simulink model "CompleteModel"  (R2020b)
settings: Solver=ode23t  StartTime=0.0  StopTime=6000  RelTol=1e-3
values from neighbouring files (symbols this model uses):
  alpha_1 = 0.5019    [Data_Parameters_CompleteModel.m]
  alpha_2 = 0.4982    [Data_Parameters_CompleteModel.m]
  Cp = 3200    [Data_Parameters_CompleteModel.m]
  D = [-D2 0 -D4 -2*D5 ... (first row only)    [Data_Parameters_CompleteModel.m]
  d = 1.5e-6    (= 1.5e-06)    [Data_Parameters_CompleteModel.m]
  D2 = 4.438e-14    [Data_Parameters_CompleteModel.m]
  D3 = 1.0024e-14    [Data_Parameters_CompleteModel.m]
  D4 = 3.8e-14    [Data_Parameters_CompleteModel.m]
  D5 = 1.75e-14    [Data_Parameters_CompleteModel.m]
  D_col = 2*A_col/(h_col+w_col)    (= 0.0193548387097)    [Data_Parameters_CompleteModel.m]
  D_L1 = [D_L11 D_L12 D_L13]    [Data_Parameters_CompleteModel.m]
  D_L2 = [D_L21 D_L22 D_L23]    [Data_Parameters_CompleteModel.m]
  D_rec = 2*A_rec/(w_rec+t_rec)    (= 0.00248962655602)    [Data_Parameters_CompleteModel.m]
  F = 96485    [Data_Parameters_CompleteModel.m]
  f_L1 = [f_L11 f_L12 f_L13]    [Data_Parameters_CompleteModel.m]
  f_L2 = [f_L21 f_L22 f_L23]    [Data_Parameters_CompleteModel.m]
  f_value = 58.91    [Data_Parameters_CompleteModel.m]
  H1 = -220000    [Data_Parameters_CompleteModel.m]
  H2 = -64000    [Data_Parameters_CompleteModel.m]
  H4 = -91200    [Data_Parameters_CompleteModel.m]
  H5 = -246800    [Data_Parameters_CompleteModel.m]
  h_col = 0.01    [Data_Parameters_CompleteModel.m]
  k0_1 = 1.6e-6    (= 1.6e-06)    [Data_Parameters_CompleteModel.m]
  k0_2 = 1.5e-4    (= 0.00015)    [Data_Parameters_CompleteModel.m]
  K_con1 = 0.35    [Data_Parameters_CompleteModel.m]
  K_con2 = 0.35    [Data_Parameters_CompleteModel.m]
  K_dec1 = 0.07    [Data_Parameters_CompleteModel.m]
  K_dec2 = 0.07    [Data_Parameters_CompleteModel.m]
  K_E1 = [K_E11 K_E12 K_E13]    [Data_Parameters_CompleteModel.m]
  K_E2 = [K_E21 K_E22 K_E23]    [Data_Parameters_CompleteModel.m]
  K_el = (df^2/(16*CKC))*(porosity^3/(1-porosity)^2)*w_el*t_el    (= 2.96777943925e-13)    [Data_Parameters_CompleteModel.m]
  K_exp1 = 0.7    [Data_Parameters_CompleteModel.m]
  K_exp2 = 0.7    [Data_Parameters_CompleteModel.m]
  K_in1 = 0.5    [Data_Parameters_CompleteModel.m]
  K_in2 = 0.5    [Data_Parameters_CompleteModel.m]
  K_inc1 = 0.68    [Data_Parameters_CompleteModel.m]
  K_inc2 = 0.68    [Data_Parameters_CompleteModel.m]
  K_out1 = 1.0    (= 1)    [Data_Parameters_CompleteModel.m]
  K_out2 = 1.0    (= 1)    [Data_Parameters_CompleteModel.m]
  K_valve1 = 0.06    [Data_Parameters_CompleteModel.m]
  K_valve2 = 0.06    [Data_Parameters_CompleteModel.m]
  Kin = 0.5    [Data_Parameters_CompleteModel.m]
  Kout = 1.0    (= 1)    [Data_Parameters_CompleteModel.m]
  L_col = 0.53    [Data_Parameters_CompleteModel.m]
  L_el = 0.3    [Data_Parameters_CompleteModel.m]
  L_L1 = [L_L11 L_L12 L_L13]    [Data_Parameters_CompleteModel.m]
  L_L2 = [L_L21 L_L22 L_L23]    [Data_Parameters_CompleteModel.m]
  L_rec = 0.02    [Data_Parameters_CompleteModel.m]
  mu = 4.928e-3    (= 0.004928)    [Data_Parameters_CompleteModel.m]
  N = 1    [Data_Parameters_CompleteModel.m]
  N_E1 = [N_E11 N_E12 N_E13]    [Data_Parameters_CompleteModel.m]
  N_E2 = [N_E21 N_E22 N_E23]    [Data_Parameters_CompleteModel.m]
  N_in1 = 2    [Data_Parameters_CompleteModel.m]
  N_in2 = 2    [Data_Parameters_CompleteModel.m]
  N_out1 = 2    [Data_Parameters_CompleteModel.m]
  N_out2 = 2    [Data_Parameters_CompleteModel.m]
  N_valves1 = 3    [Data_Parameters_CompleteModel.m]
  N_valves2 = 3    [Data_Parameters_CompleteModel.m]
  r = 0.04    [Data_Parameters_CompleteModel.m]
  R = 8.31    [Data_Parameters_CompleteModel.m]
  ro = 1354    [Data_Parameters_CompleteModel.m]
  S = 9e-4    (= 0.0009)    [Data_Parameters_CompleteModel.m]
  T = 298    [Data_Parameters_CompleteModel.m]
  t_rec = 0.00125    [Data_Parameters_CompleteModel.m]
  UpAp = 0.47    [Data_Parameters_CompleteModel.m]
  UsAs = 1.31    [Data_Parameters_CompleteModel.m]
  UtAt = 12.69    [Data_Parameters_CompleteModel.m]
  Vcell = 0.0171    [Data_Parameters_CompleteModel.m]
  Vpipe = 1.256e-3    (= 0.001256)    [Data_Parameters_CompleteModel.m]
  Vtank_Anolyte = 45e-6    (= 4.5e-05)    [Data_Parameters_CompleteModel.m]
  Vtank_Catholyte = 55.74e-6    (= 5.574e-05)    [Data_Parameters_CompleteModel.m]
  w_col = 0.3    [Data_Parameters_CompleteModel.m]
  w_rec = 0.3    [Data_Parameters_CompleteModel.m]
undefined symbols (not defined in the file or in its folder): magnitude
(part 1 of 2)
settings Model: Creator=FC_Lab  LastModifiedBy=Alejandro
settings DataIOCC: ReturnWorkspaceOutputs=off
settings DebuggingCC: ArithmeticOperatorsInVariantConditions=warning
settings SFSimCC: SimUseLocalCustomCode=off  CustomCodeUndefinedFunction=UseInterfaceOnly
settings RTWCC: RTWUseLocalCustomCode=off

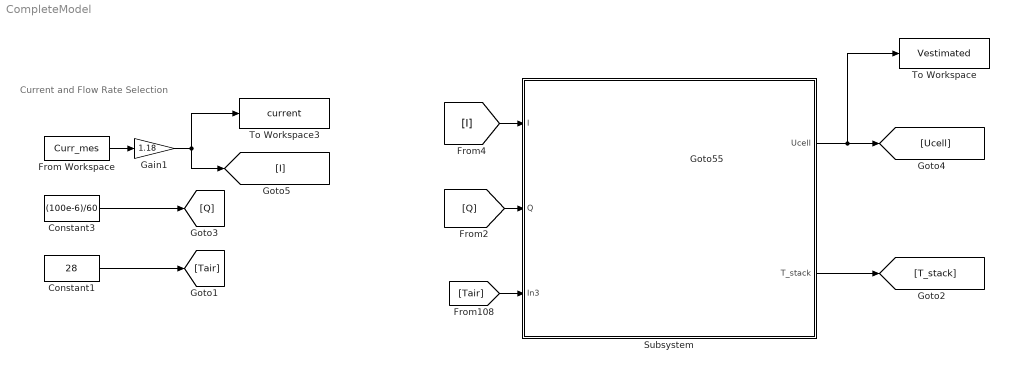
== system CompleteModel ==
  note: Current and Flow Rate Selection
  Constant1 : Constant  Value=28
  Constant3 : Constant  Value=(100e-6)/60
  From Workspace : FromWorkspace  VariableName=Curr_mes
  Gain1 : Gain  Gain=1.18
  Subsystem : Subsystem
      mask Display: image('$imagefile'); % Use "Edit Image" on toolstrip to change.
  To Workspace : ToWorkspace  VariableName=Vestimated  SampleTime=1.0
      settings: Save2DSignal=2-D array (concatenate along first dimension)
  To Workspace3 : ToWorkspace  VariableName=current  SampleTime=1.0
      settings: Save2DSignal=2-D array (concatenate along first dimension)
  wires:
  [I] -> Subsystem/1("I ")
  [Q] -> Subsystem/2(Q)
  [Tair] -> Subsystem/3(In3)
  Subsystem/1(Ucell) -> To Workspace/1, [Ucell]
  Subsystem/2(T_stack) -> [T_stack]
  Constant3/1 -> [Q]
  From Workspace/1 -> Gain1/1
  Gain1/1 -> [I], To Workspace3/1
  Constant1/1 -> [Tair]

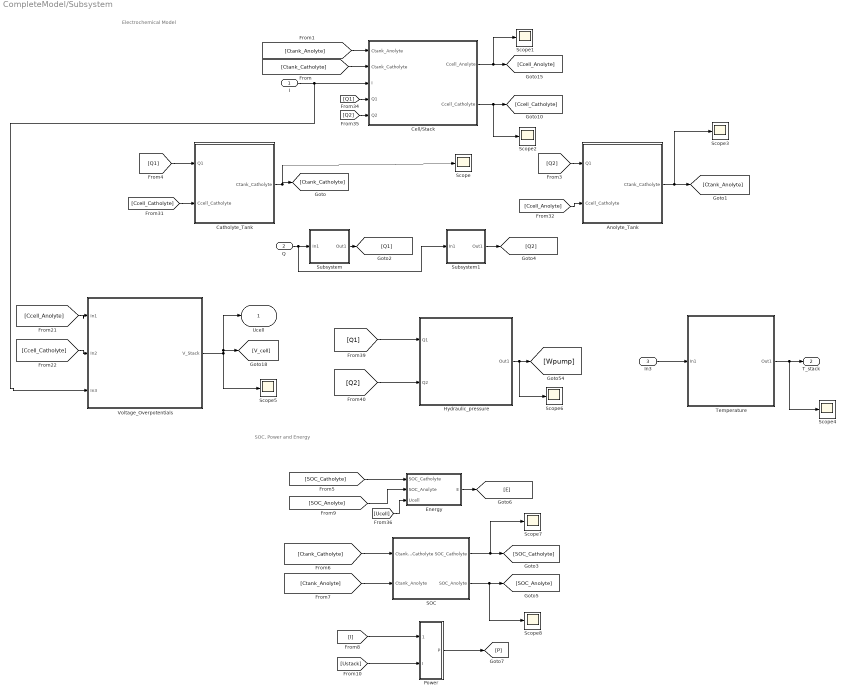
== system CompleteModel/Subsystem ==
  note: SOC, Power and Energy
  note: Electrochemical Model
  "I " : Inport
  Q : Inport  Port=2
  In3 : Inport  Port=3
  Anolyte_Tank : Subsystem  mask(Anolyte tank model){Vtank_Anolyte=55e-6, Ctankini2=5, Ctankini3=395}
      mask help: This subsystem defines the model of the anolyte tank of the redox flow batteries..
      mask Help:
      | The parameters of the block consist on:
      | 
      | Vtank_Anolyte: Volume of the anolye tank (m^3)
      | Ctankini2: Initial concentration of V2 in the anolyte tank (mol/m^3)
      | Ctankini3: Initial concentration of V3 in the anolyte tank (mol/m^3)
      mask DialogControl Container4 Prompt: References
      mask DialogControl Control2 Prompt: 1] Tang, A.; McCann, J.; Bao, J.; Skyllas-Kazacos, M. Investigation of the effect of shunt current on battery efficiency and stack temperature in vanadium redox flow battery.
      mask DialogControl Control3 Prompt: https://doi.org/10.1016/j.jpowsour.2013.05.079.
      mask DialogControl Control4 Prompt: 2] Wei, Z.; Xiong, R.; Lim, T.M.; Meng, S.; Skyllas-Kazacos, M.  Online monitoring of state of charge and1010capacity loss for vanadium redox flow battery based on autoregressive exogenous modeling.
      mask DialogControl Control5 Prompt: https://doi.org/10.1016/j.jpowsour.2018.09.028.
      mask DialogControl Container5 Prompt: Initial concentrations
      mask Display: image('$imagefile'); % Use "Edit Image" on toolstrip to change.
  Catholyte_Tank : Subsystem  mask(Catholyte tank model){Vtank_Catholyte=55e-6, Ctankini4=395, Ctankini5=5}
      mask help: This subsystem defines the model of the catholyte tank of the redox flow batteries..
      mask Help:
      | The parameters of the block consist on:
      | 
      | Vtank_Catholyte: Volume of the catholyte tank (m^3)
      | Ctankini4: Initial concentration of V4 in the cell (mol/m^3)
      | Ctankini5: Initial concentration of V5 in the cell (mol/m^3)
      mask DialogControl Container4 Prompt: References
      mask DialogControl Control2 Prompt: 1] Tang, A.; McCann, J.; Bao, J.; Skyllas-Kazacos, M. Investigation of the effect of shunt current on battery efficiency and stack temperature in vanadium redox flow battery.
      mask DialogControl Control3 Prompt: https://doi.org/10.1016/j.jpowsour.2013.05.079.
      mask DialogControl Control4 Prompt: 2] Wei, Z.; Xiong, R.; Lim, T.M.; Meng, S.; Skyllas-Kazacos, M.  Online monitoring of state of charge and1010capacity loss for vanadium redox flow battery based on autoregressive exogenous modeling.
      mask DialogControl Control5 Prompt: https://doi.org/10.1016/j.jpowsour.2018.09.028.
      mask DialogControl Container5 Prompt: Initial concentrations
      mask Display: image('$imagefile'); % Use "Edit Image" on toolstrip to change.
  Cell/Stack : Subsystem  mask(Cell-Stack model){N=1, Vcell=10e-6, S=1e-4, d=1e-4, Ccellini2=390, Ccellini3=10, Ccellini4=10, Ccellini5=390}
      mask help: This subsystem defines the model of the cell or stack of the redox flow batteries.
      mask Help:
      | The parameters of the block consist on:
      | 
      | N: Number of cells
      | Vcell: Volume of a cell (m^3)
      | S: Electrode surface (m^2)
      | d: Thickness of the membrane (m)
      | Ccellini2: Initial concentration of V2 in the cell (mol/m^3)
      | Ccellini3: Initial concentration of V3 in the cell (mol/m^3)
      | Ccellini4: Initial concentration of V4 in the cell (mol/m^3)
      | Ccellini5: Initial concentration of V5 in the cell (mol/m^3)
      mask DialogControl Container7 Prompt: References
      mask DialogControl Control6 Prompt: 1] Tang, A.; McCann, J.; Bao, J.; Skyllas-Kazacos, M. Investigation of the effect of shunt current on battery efficiency and stack temperature in vanadium redox flow battery.
      mask DialogControl Control4 Prompt: https://doi.org/10.1016/j.jpowsour.2013.05.079.
      mask DialogControl Control7 Prompt: 2] Wei, Z.; Xiong, R.; Lim, T.M.; Meng, S.; Skyllas-Kazacos, M.  Online monitoring of state of charge and1010capacity loss for vanadium redox flow battery based on autoregressive exogenous modeling.
      mask DialogControl Control8 Prompt: https://doi.org/10.1016/j.jpowsour.2018.09.028.
      mask DialogControl Container8 Prompt: Initial concentrations
      mask Display: image('$imagefile'); % Use "Edit Image" on toolstrip to change.
  Energy : Subsystem
  Hydraulic_pressure : Subsystem  mask(Hydraulic losses model){}
      mask help: THis subsystem computes the hydraulic losses due to the pressure of liquids inside the system
      mask DialogControl Container3 Prompt: References
      mask DialogControl Control2 Prompt: Tang,A.;Bao,J.;Skyllas-Kazacos,M.Studies on pressure  losses and flow rate optimization  in  vanadium  redox  flow  battery.
      mask DialogControl Control3 Prompt: https://doi.org/10.1016/j.jpowsour.2013.09.071.
      mask DialogControl Control4 Prompt: Kumar,   S.;    Jayanti,   S.Effect   of   electrode   intrusion   on   pressure   drop   and   electrochemical performance  of  an  all-vanadium  redox  flow  battery.
      mask DialogControl Control5 Prompt: https://doi.org/10.1016/j.jpowsour.2017.06.045.
      mask Display: image('$imagefile'); % Use "Edit Image" on toolstrip to change.
  Power : Subsystem
  SOC : Subsystem
  Scope{,1..8} (9 alike) : Scope
  Subsystem : Subsystem  mask(Pump model){Epump1=1}
      mask help: Model of the pump according to the manufacturer datasheet
      mask Help: Epump: Efficiency of the pump
      mask DialogControl Container4 Prompt: Manufacturer datasheet
      mask DialogControl Control2 Prompt: Model of the pump
      mask Display: image('$imagefile'); % Use "Edit Image" on toolstrip to change.
  Subsystem1 : Subsystem  mask(Pump model){Epump2=1}
      mask help: Model of the pump according to the manufacturer datasheet
      mask Help: Epump2 : Efficiency of the pump
      mask DialogControl Container4 Prompt: Manufacturer datasheet
      mask DialogControl Control2 Prompt: Model of the pump
      mask Display: image('Pump.JPG'); % Use "Edit Image" on toolstrip to change.
  Temperature : Subsystem  mask(Thermal model){}
      mask help: This subsystem presents the thermal model of the redox flow battery.
      mask DialogControl Container4 Prompt: References
      mask DialogControl Control2 Prompt: Tang,   A.;    Ting,   S.;    Bao,   J.;    Skyllas-Kazacos,   M.Thermal   modelling   and   simulation of the  all-vanadium  redox flow  battery.
      mask DialogControl Control3 Prompt: https://doi.org/10.1016/j.jpowsour.2011.11.079.
      mask DialogControl Control4 Prompt: Trovò, A.; Marini, G.; Sutto, A.; Alotto, P.; Giomo, M.; Moro, F.; Guarnieri, M.  Standby thermal model1031of a vanadium redox flow battery stack with crossover and shunt-current effects.
      mask DialogControl Control5 Prompt: https://doi.org/10.1016/j.apenergy.2019.02.067.
      mask DialogControl Control6 Prompt: Tang, A.; Bao, J.; Skyllas-Kazacos, M.  Thermal modelling of battery configuration and self-discharge reactions in vanadium redox flow battery.
      mask DialogControl Control7 Prompt: https://doi.org/10.1016/j.jpowsour.2012.06.052
      mask Display: image('$imagefile'); % Use "Edit Image" on toolstrip to change.
  Voltage_Overpotentials : Subsystem  mask(Voltage and overpotential){E0=1.33, r=0.2, Chini=2000}
      mask help: This block computes the voltage and overpotentials of the cell-stack.
      mask Help:
      | The parameters of the block consist on:
      | 
      | E0: Standard electrode potential (V)
      | r: Ohmic resistance (Ohms)
      | Chini5: Initial concentration of H in the cell (mol/m^3)
      mask DialogControl Container3 Prompt: References
      mask DialogControl Control2 Prompt: (Add text here)
      mask DialogControl Control3 Prompt: (Add text here)
      mask DialogControl Container5 Prompt: Initial concentration
      mask Display: image('$imagefile'); % Use "Edit Image" on toolstrip to change.
  Ucell : Outport
  T_stack : Outport  Port=2
  wires:
  [Ctank_Catholyte] -> Cell/Stack/2(Ctank_Catholyte)
  [Q2] -> Anolyte_Tank/1(Q1)
  [Ccell_Anolyte] -> Anolyte_Tank/2(Ccell_Catholyte)
  [Ustack] -> Power/2(I)
  [SOC_Catholyte] -> Energy/1(SOC_Catholyte)
  Catholyte_Tank/1(Ctank_Catholyte) -> Scope/1, [Ctank_Catholyte]
  Cell/Stack/1(Ccell_Anolyte) -> Scope1/1, [Ccell_Anolyte]
  SOC/2(SOC_Anolyte) -> Scope8/1, [SOC_Anolyte]
  [Q2] -> Cell/Stack/5(Q2)
  [Q1] -> Cell/Stack/4(Q1)
  Energy/1(E) -> [E]
  Cell/Stack/2(Ccell_Catholyte) -> Scope2/1, [Ccell_Catholyte]
  Power/1("P ") -> [P]
  [Ccell_Catholyte] -> Catholyte_Tank/2(Ccell_Catholyte)
  [Ucell] -> Energy/3("Ucell ")
  [Ctank_Anolyte] -> Cell/Stack/1(Ctank_Anolyte)
  [SOC_Anolyte] -> Energy/2(SOC_Anolyte)
  [Ctank_Anolyte] -> SOC/2(Ctank_Anolyte)
  SOC/1(SOC_Catholyte) -> Scope7/1, [SOC_Catholyte]
  [Ctank_Catholyte] -> SOC/1(Ctank_Catholyte)
  [I] -> Power/1(Ustack)
  Anolyte_Tank/1(Ctank_Catholyte) -> Scope3/1, [Ctank_Anolyte]
  "I "/1 -> Voltage_Overpotentials/3(In3), Cell/Stack/3("I ")
  [Q1] -> Catholyte_Tank/1(Q1)
  Subsystem/1(Out1) -> [Q1]
  Subsystem1/1(Out1) -> [Q2]
  Q/1 -> Subsystem1/1(In1), Subsystem/1(In1)
  [Ccell_Anolyte] -> Voltage_Overpotentials/1(In1)
  [Ccell_Catholyte] -> Voltage_Overpotentials/2(In2)
  Voltage_Overpotentials/1(V_Stack) -> Ucell/1, [V_cell], Scope5/1
  [Q1] -> Hydraulic_pressure/1(Q1)
  [Q2] -> Hydraulic_pressure/2(Q2)
  Hydraulic_pressure/1(Out1) -> Scope6/1, [Wpump]
  In3/1 -> Temperature/1(In1)
  Temperature/1(Out1) -> Scope4/1, T_stack/1

== system CompleteModel/Subsystem/Anolyte_Tank ==
  Q1 : Inport
  Ccell_Catholyte : Inport  Port=2
  Gain1 : Gain
  Gain13 : Gain  Gain=1/Vtank_Anolyte
  Integrator Limited4 : Integrator  InitialCondition=[Ctankini2 Ctankini3]  LimitOutput=on  UpperSaturationLimit=400  LowerSaturationLimit=0.001
  Product15 : Product
  Product16 : Product
  Sum12 : Sum  Inputs=|+-
  Ctank_Catholyte : Outport  VectorParamsAs1DForOutWhenUnconnected=off
  wires:
  Gain13/1 -> Integrator Limited4/1
  Sum12/1 -> Gain1/1
  Q1/1 -> Product16/1, Product15/1
  Integrator Limited4/1 -> Ctank_Catholyte/1, Product16/2
  Product15/1 -> Sum12/1
  Product16/1 -> Sum12/2
  Ccell_Catholyte/1 -> Product15/2
  Gain1/1 -> Gain13/1

== system CompleteModel/Subsystem/Catholyte_Tank ==
  Q1 : Inport
  Ccell_Catholyte : Inport  Port=2
  Gain1 : Gain
  Gain13 : Gain  Gain=1/Vtank_Catholyte
  Integrator Limited4 : Integrator  InitialCondition=[Ctankini4 Ctankini5]  LimitOutput=on  UpperSaturationLimit=400  LowerSaturationLimit=0.001
  Product15 : Product
  Product16 : Product
  Sum12 : Sum  Inputs=|+-
  Ctank_Catholyte : Outport  VectorParamsAs1DForOutWhenUnconnected=off
  wires:
  Gain13/1 -> Integrator Limited4/1
  Sum12/1 -> Gain1/1
  Q1/1 -> Product16/1, Product15/1
  Integrator Limited4/1 -> Ctank_Catholyte/1, Product16/2
  Product15/1 -> Sum12/1
  Product16/1 -> Sum12/2
  Ccell_Catholyte/1 -> Product15/2
  Gain1/1 -> Gain13/1

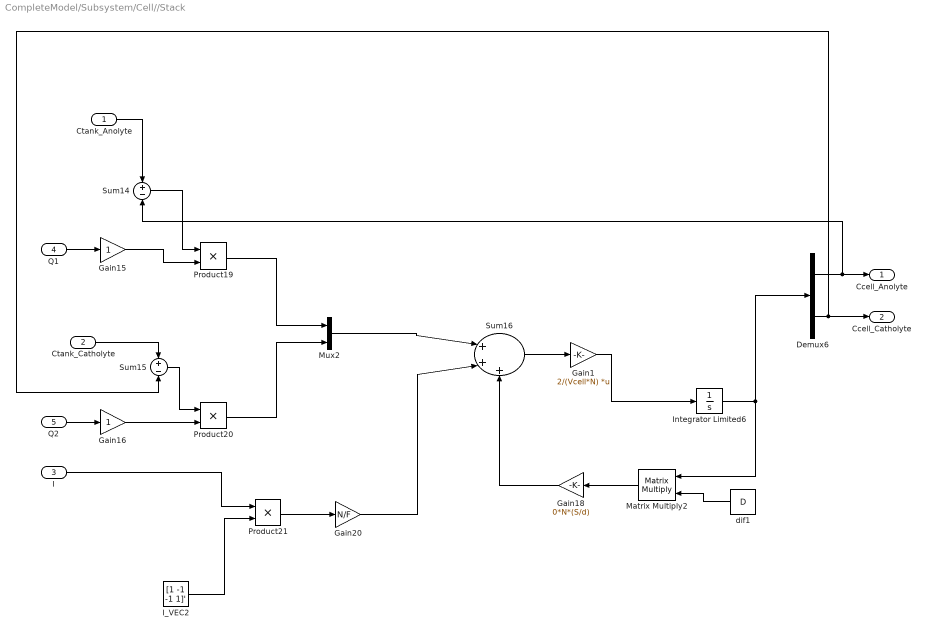
== system CompleteModel/Subsystem/Cell//Stack ==
  Ctank_Anolyte : Inport
  Ctank_Catholyte : Inport  Port=2
  "I " : Inport  Port=3
  Q1 : Inport  Port=4
  Q2 : Inport  Port=5
  Demux6 : Demux  Outputs=2
  Gain1 : Gain  Gain=2/(Vcell*N)  Multiplication=Matrix(K*u)
  Gain15 : Gain
  Gain16 : Gain
  Gain18 : Gain  Gain=0*N*(S/d)
  Gain20 : Gain  Gain=N/F
  I_VEC2 : Constant  Value=[1 -1 -1 1]'
  Integrator Limited6 : Integrator  InitialCondition=[Ccellini2 Ccellini3 Ccellini4 Ccellini5]  LimitOutput=on  UpperSaturationLimit=400  LowerSaturationLimit=0.001
  Matrix Multiply2 : Product  Multiplication=Matrix(*)
  Mux2 : Mux  Inputs=2
  Product19 : Product
  Product20 : Product
  Product21 : Product
  Sum14 : Sum  Inputs=+-
  Sum15 : Sum  Inputs=+-
  Sum16 : Sum  Inputs=|+++
  dif1 : Constant  Value=D
  Ccell_Anolyte : Outport  VectorParamsAs1DForOutWhenUnconnected=off
  Ccell_Catholyte : Outport  Port=2  VectorParamsAs1DForOutWhenUnconnected=off
  wires:
  Gain18/1 -> Sum16/3
  Ctank_Anolyte/1 -> Sum14/1
  Gain20/1 -> Sum16/2
  "I "/1 -> Product21/1
  Integrator Limited6/1 -> Matrix Multiply2/1, Demux6/1
  Sum16/1 -> Gain1/1
  Gain15/1 -> Product19/2
  Sum14/1 -> Product19/1
  Product21/1 -> Gain20/1
  I_VEC2/1 -> Product21/2
  Product19/1 -> Mux2/1
  Sum15/1 -> Product20/1
  Gain16/1 -> Product20/2
  Q1/1 -> Gain15/1
  Matrix Multiply2/1 -> Gain18/1
  dif1/1 -> Matrix Multiply2/2
  Product20/1 -> Mux2/2
  Ctank_Catholyte/1 -> Sum15/1
  Q2/1 -> Gain16/1
  Mux2/1 -> Sum16/1
  Gain1/1 -> Integrator Limited6/1
  Demux6/1 -> Sum14/2, Ccell_Anolyte/1
  Demux6/2 -> Ccell_Catholyte/1, Sum15/2

== system CompleteModel/Subsystem/Energy ==
  SOC_Catholyte : Inport
  SOC_Anolyte : Inport  Port=2
  "Ucell " : Inport  Port=3
  Add : Sum
  Add1 : Sum
  Constant1 : Constant  Value=Vtank_Catholyte
  Constant2 : Constant  Value=F
  Constant3 : Constant  Value=Vtank_Anolyte
  Constant4 : Constant  Value=2000
  Divide11 : Product  Inputs=**
  Divide9 : Product  Inputs=****
  Gain : Gain  Gain=0.5
  Gain1 : Gain  Gain=0.5
  E : Outport  VectorParamsAs1DForOutWhenUnconnected=off
  wires:
  SOC_Anolyte/1 -> Add/2
  Constant2/1 -> Divide9/1
  Divide9/1 -> Divide11/1
  Gain/1 -> Divide9/2
  Add1/1 -> Gain1/1
  Divide11/1 -> E/1
  "Ucell "/1 -> Divide11/2
  Add/1 -> Gain/1
  SOC_Catholyte/1 -> Add/1
  Constant1/1 -> Add1/1
  Constant3/1 -> Add1/2
  Gain1/1 -> Divide9/3
  Constant4/1 -> Divide9/4

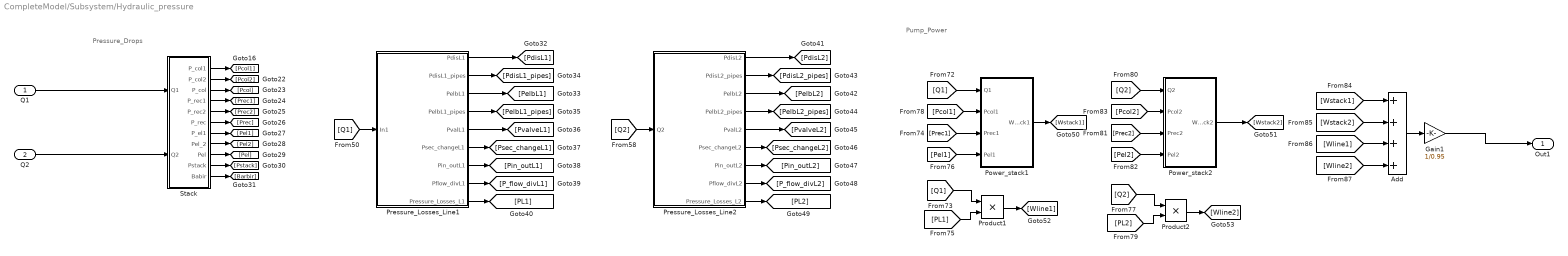
== system CompleteModel/Subsystem/Hydraulic_pressure ==
  note: Pump_Power
  note: Pressure_Drops
  Q1 : Inport
  Q2 : Inport  Port=2
  Add : Sum  Inputs=++++
  Gain1 : Gain  Gain=1/0.95
  Power_stack1 : Subsystem
  Power_stack2 : Subsystem
  Pressure_Losses_Line1 : Subsystem
  Pressure_Losses_Line2 : Subsystem
  Product1 : Product
  Product2 : Product
  Stack : Subsystem
  Out1 : Outport
  wires:
  Pressure_Losses_Line1/7(Pin_outL1) -> [Pin_outL1]
  [Prec1] -> Power_stack1/3(Prec1)
  Pressure_Losses_Line2/2(PdisL2_pipes) -> [PdisL2_pipes]
  [Pcol1] -> Power_stack1/2(Pcol1)
  Stack/2(P_col2) -> [Pcol2]
  Pressure_Losses_Line2/5(PvalL2) -> [PvalveL2]
  Pressure_Losses_Line2/6(Psec_changeL2) -> [Psec_changeL2]
  Power_stack1/1(Wstack1) -> [Wstack1]
  [Q2] -> Pressure_Losses_Line2/1(Q2)
  [Q1] -> Pressure_Losses_Line1/1(In1)
  Add/1 -> Gain1/1
  [Pel1] -> Power_stack1/4(Pel1)
  [Wline2] -> Add/4
  Pressure_Losses_Line2/8(Pflow_divL2) -> [P_flow_divL2]
  Stack/8(Pel_2) -> [Pel2]
  Pressure_Losses_Line2/1(PdisL2) -> [PdisL2]
  Gain1/1 -> Out1/1
  [Wstack1] -> Add/1
  Stack/10(Pstack) -> [Pstack]
  Q1/1 -> Stack/1(Q1)
  Stack/7(P_el1) -> [Pel1]
  Pressure_Losses_Line1/8(Pflow_divL1) -> [P_flow_divL1]
  [Wline1] -> Add/3
  Pressure_Losses_Line2/4(PelbL2_pipes) -> [PelbL2_pipes]
  [PL2] -> Product2/2
  Pressure_Losses_Line1/5(PvalL1) -> [PvalveL1]
  Stack/9(Pel) -> [Pel]
  [Q2] -> Power_stack2/1(Q2)
  Stack/11(Babir) -> [Barbir]
  [PL1] -> Product1/2
  [Q2] -> Product2/1
  [Pel2] -> Power_stack2/4(Pel2)
  Pressure_Losses_Line1/1(PdisL1) -> [PdisL1]
  Pressure_Losses_Line1/4(PelbL1_pipes) -> [PelbL1_pipes]
  Product1/1 -> [Wline1]
  Pressure_Losses_Line1/3(PelbL1) -> [PelbL1]
  Stack/1("P_col1 ") -> [Pcol1]
  [Wstack2] -> Add/2
  Stack/3(P_col) -> [Pcol]
  Stack/6(P_rec) -> [Prec]
  Product2/1 -> [Wline2]
  [Q1] -> Power_stack1/1(Q1)
  Pressure_Losses_Line1/2(PdisL1_pipes) -> [PdisL1_pipes]
  Stack/4(P_rec1) -> [Prec1]
  Power_stack2/1(Wstack2) -> [Wstack2]
  Pressure_Losses_Line1/6(Psec_changeL1) -> [Psec_changeL1]
  [Q1] -> Product1/1
  Q2/1 -> Stack/2(Q2)
  [Prec2] -> Power_stack2/3(Prec2)
  Pressure_Losses_Line2/7(Pin_outL2) -> [Pin_outL2]
  Pressure_Losses_Line2/9(Pressure_Losses_L2) -> [PL2]
  Stack/5(P_rec2) -> [Prec2]
  [Pcol2] -> Power_stack2/2(Pcol2)
  Pressure_Losses_Line2/3(PelbL2) -> [PelbL2]
  Pressure_Losses_Line1/9(Pressure_Losses_L1) -> [PL1]

== system CompleteModel/Subsystem/Power ==
  Ustack : Inport
  I : Inport  Port=2
  Divide11 : Product  Inputs=**
  "P " : Outport  VectorParamsAs1DForOutWhenUnconnected=off
  wires:
  Ustack/1 -> Divide11/1
  Divide11/1 -> "P "/1
  I/1 -> Divide11/2

== system CompleteModel/Subsystem/SOC ==
  Ctank_Catholyte : Inport
  Ctank_Anolyte : Inport  Port=2
  Demux1 : Demux  Outputs=2
  Demux2 : Demux  Outputs=2
  Divide6 : Product  Inputs=*/
  Divide7 : Product  Inputs=*/
  Sum10 : Sum  Inputs=|++
  Sum9 : Sum  Inputs=|++
  SOC_Catholyte : Outport  VectorParamsAs1DForOutWhenUnconnected=off
  SOC_Anolyte : Outport  Port=2  VectorParamsAs1DForOutWhenUnconnected=off
  wires:
  Ctank_Catholyte/1 -> Demux1/1
  Sum10/1 -> Divide7/2
  Demux2/2 -> Divide7/1, Sum10/2
  Sum9/1 -> Divide6/2
  Divide7/1 -> SOC_Anolyte/1
  Demux1/1 -> Sum9/1, Divide6/1
  Demux2/1 -> Sum10/1
  Demux1/2 -> Sum9/2
  Divide6/1 -> SOC_Catholyte/1
  Ctank_Anolyte/1 -> Demux2/1

== system CompleteModel/Subsystem/Subsystem ==
  In1 : Inport
  Gain : Gain  Gain=Epump1
  Out1 : Outport
  wires:
  In1/1 -> Gain/1
  Gain/1 -> Out1/1

== system CompleteModel/Subsystem/Subsystem1 ==
  In1 : Inport
  Gain : Gain  Gain=Epump2
  Out1 : Outport
  wires:
  In1/1 -> Gain/1
  Gain/1 -> Out1/1

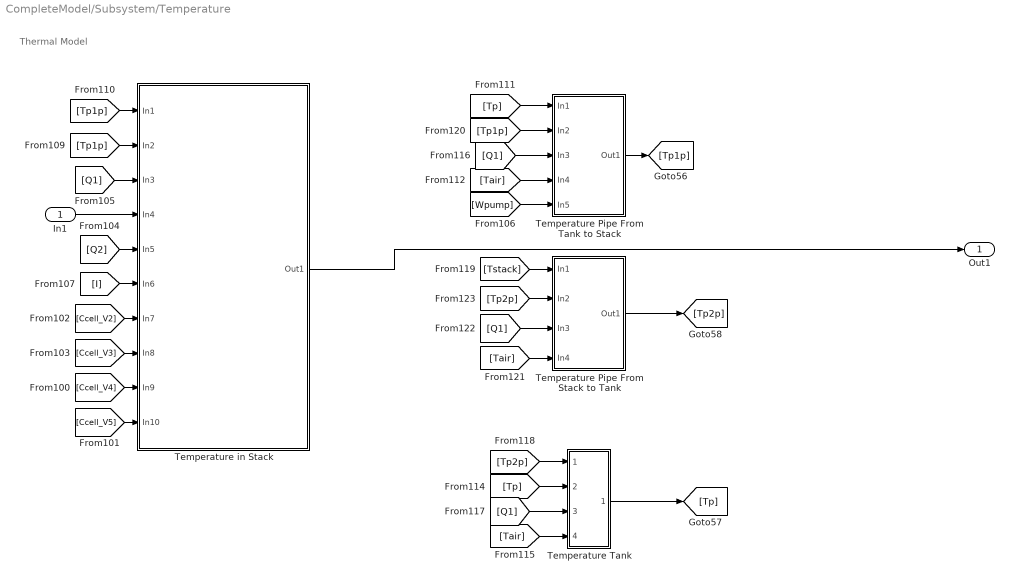
== system CompleteModel/Subsystem/Temperature ==
  note: Thermal Model
  In1 : Inport
  Temperature Tank : Subsystem
  Temperature Pipe From Stack to Tank : Subsystem
  "Temperature Pipe From Tank to Stack " : Subsystem
  Temperature in Stack : Subsystem
  Out1 : Outport
  wires:
  [Ccell_V4] -> Temperature in Stack/9(In9)
  [Q1] -> "Temperature Pipe From Tank to Stack "/3(In3)
  [Ccell_V3] -> Temperature in Stack/8(In8)
  [Tp1p] -> Temperature in Stack/1(In1)
  [Q2] -> Temperature in Stack/5(In5)
  [Tair] -> Temperature Pipe From Stack to Tank/4(In4)
  [Tp2p] -> Temperature Pipe From Stack to Tank/2(In2)
  [Ccell_V2] -> Temperature in Stack/7(In7)
  [Wpump] -> "Temperature Pipe From Tank to Stack "/5(In5)
  [Tp] -> Temperature Tank/2(In2)
  [Q1] -> Temperature Pipe From Stack to Tank/3(In3)
  [Ccell_V5] -> Temperature in Stack/10(In10)
  [Tair] -> "Temperature Pipe From Tank to Stack "/4(In4)
  [Tp2p] -> Temperature Tank/1(In1)
  [Tstack] -> Temperature Pipe From Stack to Tank/1(In1)
  [Q1] -> Temperature Tank/3(In3)
  [Tp1p] -> Temperature in Stack/2(In2)
  [I] -> Temperature in Stack/6(In6)
  [Tair] -> Temperature Tank/4(In4)
  Temperature Pipe From Stack to Tank/1(Out1) -> [Tp2p]
  [Tp1p] -> "Temperature Pipe From Tank to Stack "/2(In2)
  "Temperature Pipe From Tank to Stack "/1(Out1) -> [Tp1p]
  [Tp] -> "Temperature Pipe From Tank to Stack "/1(In1)
  Temperature Tank/1(Out1) -> [Tp]
  [Q1] -> Temperature in Stack/3(In3)
  Temperature in Stack/1(Out1) -> Out1/1
  In1/1 -> Temperature in Stack/4(In4)

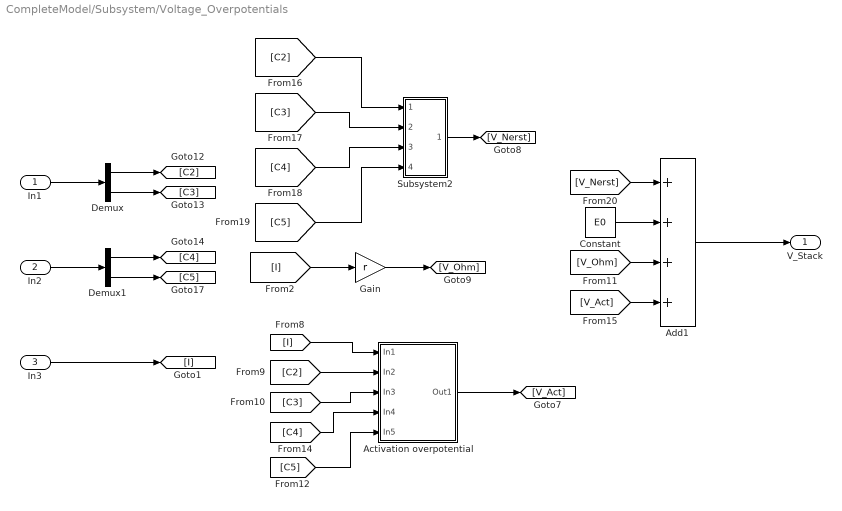
== system CompleteModel/Subsystem/Voltage_Overpotentials ==
  In1 : Inport
  In2 : Inport  Port=2
  In3 : Inport  Port=3
  Activation overpotential : Subsystem
  Add1 : Sum  Inputs=++++
  Constant : Constant  Value=E0
  Demux : Demux  Outputs=2
  Demux1 : Demux  Outputs=2
  Gain : Gain  Gain=r
  Subsystem2 : Subsystem
  V_Stack : Outport
  wires:
  Demux/2 -> [C3]
  Demux1/2 -> [C5]
  Demux1/1 -> [C4]
  Demux/1 -> [C2]
  In1/1 -> Demux/1
  In2/1 -> Demux1/1
  In3/1 -> [I]
  [I] -> Activation overpotential/1(In1)
  Constant/1 -> Add1/2
  Activation overpotential/1(Out1) -> [V_Act]
  [C5] -> Activation overpotential/5(In5)
  [I] -> Gain/1
  Gain/1 -> [V_Ohm]
  [C4] -> Activation overpotential/4(In4)
  [C2] -> Activation overpotential/2(In2)
  [V_Act] -> Add1/4
  [C4] -> Subsystem2/3(In3)
  [V_Ohm] -> Add1/3
  [V_Nerst] -> Add1/1
  [C3] -> Activation overpotential/3(In3)
  Add1/1 -> V_Stack/1
  Subsystem2/1(Out1) -> [V_Nerst]
  [C3] -> Subsystem2/2(In2)
  [C5] -> Subsystem2/4(In4)
  [C2] -> Subsystem2/1(In1)

== system CompleteModel/Subsystem/Hydraulic_pressure/Power_stack1 ==
  Q1 : Inport
  Pcol1 : Inport  Port=2
  Prec1 : Inport  Port=3
  Pel1 : Inport  Port=4
  Add : Sum  Inputs=+++
  Product : Product
  Product1 : Product
  Product2 : Product
  Wstack1 : Outport  VectorParamsAs1DForOutWhenUnconnected=off
  wires:
  Prec1/1 -> Product/2
  Pel1/1 -> Product2/1
  Q1/1 -> Product/1, Product2/2, Product1/1
  Product2/1 -> Add/3
  Add/1 -> Wstack1/1
  Pcol1/1 -> Product1/2
  Product/1 -> Add/2
  Product1/1 -> Add/1

== system CompleteModel/Subsystem/Hydraulic_pressure/Power_stack2 ==
  Q2 : Inport
  Pcol2 : Inport  Port=2
  Prec2 : Inport  Port=3
  Pel2 : Inport  Port=4
  Add : Sum  Inputs=+++
  Product : Product
  Product1 : Product
  Product2 : Product
  Wstack2 : Outport  VectorParamsAs1DForOutWhenUnconnected=off
  wires:
  Prec2/1 -> Product/2
  Pel2/1 -> Product2/1
  Q2/1 -> Product/1, Product2/2, Product1/1
  Product2/1 -> Add/3
  Add/1 -> Wstack2/1
  Pcol2/1 -> Product1/2
  Product/1 -> Add/2
  Product1/1 -> Add/1

== system CompleteModel/Subsystem/Hydraulic_pressure/Pressure_Losses_Line1 ==
  In1 : Inport
  Add : Sum  Inputs=++++++
  Elbows_Losses : Subsystem
  Flow_Division_Losses : Subsystem
  Input_Output_Losses : Subsystem
  Pipes_Distributed_Losses : Subsystem
  Section_Change_Losses : Subsystem
  Valves_Losses : Subsystem
  PdisL1 : Outport  VectorParamsAs1DForOutWhenUnconnected=off
  PdisL1_pipes : Outport  Port=2  VectorParamsAs1DForOutWhenUnconnected=off
  PelbL1 : Outport  Port=3  VectorParamsAs1DForOutWhenUnconnected=off
  PelbL1_pipes : Outport  Port=4  VectorParamsAs1DForOutWhenUnconnected=off
  PvalL1 : Outport  Port=5  VectorParamsAs1DForOutWhenUnconnected=off
  Psec_changeL1 : Outport  Port=6  VectorParamsAs1DForOutWhenUnconnected=off
  Pin_outL1 : Outport  Port=7  VectorParamsAs1DForOutWhenUnconnected=off
  Pflow_divL1 : Outport  Port=8  VectorParamsAs1DForOutWhenUnconnected=off
  Pressure_Losses_L1 : Outport  Port=9  VectorParamsAs1DForOutWhenUnconnected=off
  wires:
  In1/1 -> Elbows_Losses/1(Q1), Valves_Losses/1(Q1), Section_Change_Losses/1(Q1), Input_Output_Losses/1(Q1), Flow_Division_Losses/1(Q1), Pipes_Distributed_Losses/1("Q1 ")
  Section_Change_Losses/1(Psec_change) -> Add/4, Psec_changeL1/1
  Pipes_Distributed_Losses/1(Pdis_L1) -> Add/1, PdisL1/1
  Valves_Losses/1(Pval) -> Add/3, PvalL1/1
  Pipes_Distributed_Losses/2(Pdis_L1_pipes) -> PdisL1_pipes/1
  Elbows_Losses/2(Pelb_pipes) -> PelbL1_pipes/1
  Elbows_Losses/1(Pelb) -> Add/2, PelbL1/1
  Flow_Division_Losses/1(Pflow_div) -> Add/6, Pflow_divL1/1
  Input_Output_Losses/1(Pin_out) -> Add/5, Pin_outL1/1
  Add/1 -> Pressure_Losses_L1/1

== system CompleteModel/Subsystem/Hydraulic_pressure/Pressure_Losses_Line2 ==
  Q2 : Inport
  Add : Sum  Inputs=++++++
  Elbows_Losses : Subsystem
  Flow_Division_Losses : Subsystem
  Input_Output_Losses : Subsystem
  Pipes_Distributed_Losses : Subsystem
  Section_Change_Losses : Subsystem
  Valves_Losses : Subsystem
  PdisL2 : Outport  VectorParamsAs1DForOutWhenUnconnected=off
  PdisL2_pipes : Outport  Port=2  VectorParamsAs1DForOutWhenUnconnected=off
  PelbL2 : Outport  Port=3  VectorParamsAs1DForOutWhenUnconnected=off
  PelbL2_pipes : Outport  Port=4  VectorParamsAs1DForOutWhenUnconnected=off
  PvalL2 : Outport  Port=5  VectorParamsAs1DForOutWhenUnconnected=off
  Psec_changeL2 : Outport  Port=6  VectorParamsAs1DForOutWhenUnconnected=off
  Pin_outL2 : Outport  Port=7  VectorParamsAs1DForOutWhenUnconnected=off
  Pflow_divL2 : Outport  Port=8  VectorParamsAs1DForOutWhenUnconnected=off
  Pressure_Losses_L2 : Outport  Port=9  VectorParamsAs1DForOutWhenUnconnected=off
  wires:
  Q2/1 -> Elbows_Losses/1(Q2), Valves_Losses/1(Q2), Section_Change_Losses/1(Q2), Input_Output_Losses/1(Q2), Flow_Division_Losses/1(Q2), Pipes_Distributed_Losses/1(Q2)
  Section_Change_Losses/1(Psec_change) -> Add/4, Psec_changeL2/1
  Pipes_Distributed_Losses/1(Pdis) -> Add/1, PdisL2/1
  Valves_Losses/1(Pval) -> Add/3, PvalL2/1
  Pipes_Distributed_Losses/2(Pdis_pipes) -> PdisL2_pipes/1
  Elbows_Losses/2(Pelb_pipes) -> PelbL2_pipes/1
  Elbows_Losses/1(Pelb) -> Add/2, PelbL2/1
  Flow_Division_Losses/1(Pflow_div) -> Add/6, Pflow_divL2/1
  Input_Output_Losses/1(Pin_out) -> Add/5, Pin_outL2/1
  Add/1 -> Pressure_Losses_L2/1

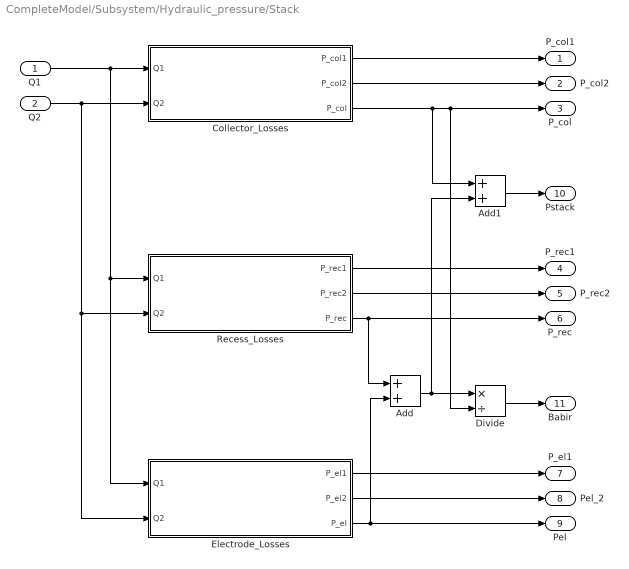
== system CompleteModel/Subsystem/Hydraulic_pressure/Stack ==
  Q1 : Inport
  Q2 : Inport  Port=2
  Add : Sum
  Add1 : Sum
  Collector_Losses : Subsystem
  Divide : Product  Inputs=*/
  Electrode_Losses : Subsystem
  Recess_Losses : Subsystem
  "P_col1 " : Outport  VectorParamsAs1DForOutWhenUnconnected=off
  P_col2 : Outport  Port=2  VectorParamsAs1DForOutWhenUnconnected=off
  P_col : Outport  Port=3  VectorParamsAs1DForOutWhenUnconnected=off
  P_rec1 : Outport  Port=4  VectorParamsAs1DForOutWhenUnconnected=off
  P_rec2 : Outport  Port=5  VectorParamsAs1DForOutWhenUnconnected=off
  P_rec : Outport  Port=6  VectorParamsAs1DForOutWhenUnconnected=off
  P_el1 : Outport  Port=7  VectorParamsAs1DForOutWhenUnconnected=off
  Pel_2 : Outport  Port=8  VectorParamsAs1DForOutWhenUnconnected=off
  Pel : Outport  Port=9  VectorParamsAs1DForOutWhenUnconnected=off
  Pstack : Outport  Port=10  VectorParamsAs1DForOutWhenUnconnected=off
  Babir : Outport  Port=11  VectorParamsAs1DForOutWhenUnconnected=off
  wires:
  Collector_Losses/3(P_col) -> Add1/1, Divide/2, P_col/1
  Recess_Losses/2(P_rec2) -> P_rec2/1
  Q2/1 -> Electrode_Losses/2(Q2), Recess_Losses/2(Q2), Collector_Losses/2(Q2)
  Electrode_Losses/3(P_el) -> Add/2, Pel/1
  Q1/1 -> Electrode_Losses/1(Q1), Recess_Losses/1(Q1), Collector_Losses/1(Q1)
  Electrode_Losses/1(P_el1) -> P_el1/1
  Recess_Losses/3(P_rec) -> Add/1, P_rec/1
  Recess_Losses/1(P_rec1) -> P_rec1/1
  Electrode_Losses/2(P_el2) -> Pel_2/1
  Collector_Losses/2(P_col2) -> P_col2/1
  Collector_Losses/1(P_col1) -> "P_col1 "/1
  Add/1 -> Add1/2, Divide/1
  Divide/1 -> Babir/1
  Add1/1 -> Pstack/1

== system CompleteModel/Subsystem/Temperature/Temperature Tank ==
  In1 : Inport
  In2 : Inport  Port=2
  In3 : Inport  Port=3
  In4 : Inport  Port=4
  Add10 : Sum  Inputs=+-
  Add7 : Sum
  Add9 : Sum  Inputs=+-
  Divide4 : Product  Inputs=**
  Gain14 : Gain  Gain=UtAt
  Gain15 : Gain  Gain=1/(Cp*ro*Vtank_Catholyte)
  Gain16 : Gain  Gain=Cp*ro
  Integrator9 : Integrator  InitialCondition=20
  Out1 : Outport
  wires:
  Divide4/1 -> Add7/1
  Add9/1 -> Gain16/1
  Gain14/1 -> Add7/2
  Add7/1 -> Gain15/1
  Gain15/1 -> Integrator9/1
  In2/1 -> Add10/2, Add9/2
  Gain16/1 -> Divide4/1
  In3/1 -> Divide4/2
  Add10/1 -> Gain14/1
  In1/1 -> Add9/1
  In4/1 -> Add10/1
  Integrator9/1 -> Out1/1

== system CompleteModel/Subsystem/Temperature/Temperature Pipe From Stack to Tank ==
  In1 : Inport
  In2 : Inport  Port=2
  In3 : Inport  Port=3
  In4 : Inport  Port=4
  Add11 : Sum
  Add12 : Sum  Inputs=+-
  Add13 : Sum  Inputs=+-
  Divide5 : Product  Inputs=**
  Gain17 : Gain  Gain=UpAp
  Gain18 : Gain  Gain=1/(Cp*ro*Vpipe)
  Gain19 : Gain  Gain=Cp*ro
  Integrator2 : Integrator
  Out1 : Outport
  wires:
  In2/1 -> Add13/2, Add12/2
  Gain18/1 -> Integrator2/1
  Gain17/1 -> Add11/2
  Add13/1 -> Gain17/1
  Divide5/1 -> Add11/1
  Add11/1 -> Gain18/1
  Add12/1 -> Gain19/1
  Gain19/1 -> Divide5/1
  In1/1 -> Add12/1
  In3/1 -> Divide5/2
  Integrator2/1 -> Out1/1
  In4/1 -> Add13/1

== system CompleteModel/Subsystem/Temperature/Temperature Pipe From Tank to Stack  ==
  In1 : Inport
  In2 : Inport  Port=2
  In3 : Inport  Port=3
  In4 : Inport  Port=4
  In5 : Inport  Port=5
  Add5 : Sum  Inputs=+++
  Add6 : Sum  Inputs=+-
  Add8 : Sum  Inputs=+-
  Divide3 : Product  Inputs=**
  Gain11 : Gain  Gain=UpAp
  Gain12 : Gain  Gain=1/(Cp*ro*Vpipe)
  Gain13 : Gain  Gain=Cp*ro
  Integrator8 : Integrator
  Out1 : Outport
  wires:
  Gain13/1 -> Divide3/1
  In3/1 -> Divide3/2
  Add6/1 -> Gain13/1
  Add8/1 -> Gain11/1
  Gain12/1 -> Integrator8/1
  Divide3/1 -> Add5/1
  In2/1 -> Add8/2, Add6/2
  Gain11/1 -> Add5/2
  Add5/1 -> Gain12/1
  In5/1 -> Add5/3
  In4/1 -> Add8/1
  In1/1 -> Add6/1
  Integrator8/1 -> Out1/1

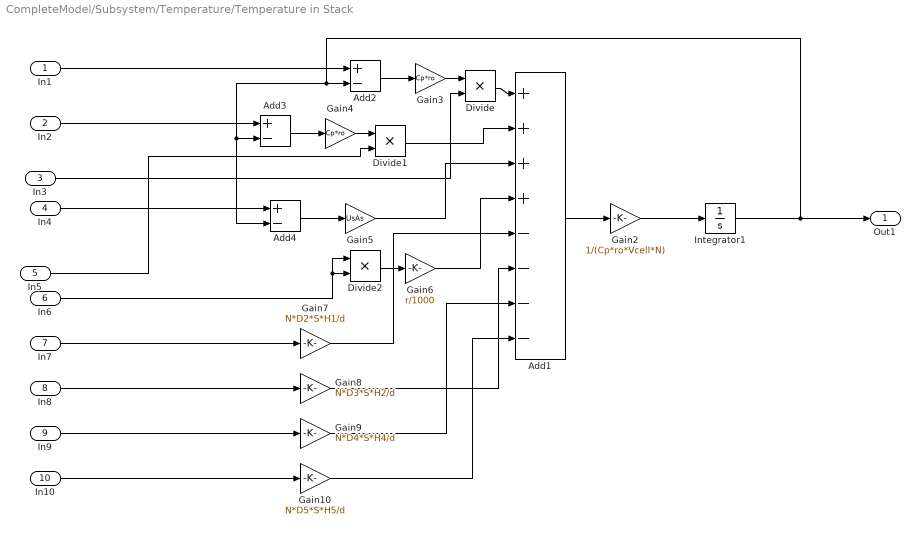
== system CompleteModel/Subsystem/Temperature/Temperature in Stack ==
  In1 : Inport
  In2 : Inport  Port=2
  In3 : Inport  Port=3
  In4 : Inport  Port=4
  In5 : Inport  Port=5
  In6 : Inport  Port=6
  In7 : Inport  Port=7
  In8 : Inport  Port=8
  In9 : Inport  Port=9
  In10 : Inport  Port=10
  Add1 : Sum  Inputs=++++----
  Add2 : Sum  Inputs=+-
  Add3 : Sum  Inputs=+-
  Add4 : Sum  Inputs=+-
  Divide : Product  Inputs=**
  Divide1 : Product  Inputs=**
  Divide2 : Product  Inputs=**
  Gain10 : Gain  Gain=N*D5*S*H5/d
  Gain2 : Gain  Gain=1/(Cp*ro*Vcell*N)
  Gain3 : Gain  Gain=Cp*ro
  Gain4 : Gain  Gain=Cp*ro
  Gain5 : Gain  Gain=UsAs
  Gain6 : Gain  Gain=r/1000
  Gain7 : Gain  Gain=N*D2*S*H1/d
  Gain8 : Gain  Gain=N*D3*S*H2/d
  Gain9 : Gain  Gain=N*D4*S*H4/d
  Integrator1 : Integrator  InitialCondition=20
  Out1 : Outport
  wires:
  Gain9/1 -> Add1/7
  Integrator1/1 -> Out1/1, Add2/2, Add4/2, Add3/2
  Gain2/1 -> Integrator1/1
  Gain8/1 -> Add1/6
  Add1/1 -> Gain2/1
  Divide/1 -> Add1/1
  In7/1 -> Gain7/1
  Gain10/1 -> Add1/8
  Gain7/1 -> Add1/5
  Divide2/1 -> Gain6/1
  Add2/1 -> Gain3/1
  In5/1 -> Divide1/2
  Gain3/1 -> Divide/1
  In6/1 -> Divide2/1, Divide2/2
  Add3/1 -> Gain4/1
  In3/1 -> Divide/2
  Gain6/1 -> Add1/4
  Divide1/1 -> Add1/2
  Gain4/1 -> Divide1/1
  Add4/1 -> Gain5/1
  Gain5/1 -> Add1/3
  In8/1 -> Gain8/1
  In9/1 -> Gain9/1
  In4/1 -> Add4/1
  In1/1 -> Add2/1
  In2/1 -> Add3/1
  In10/1 -> Gain10/1

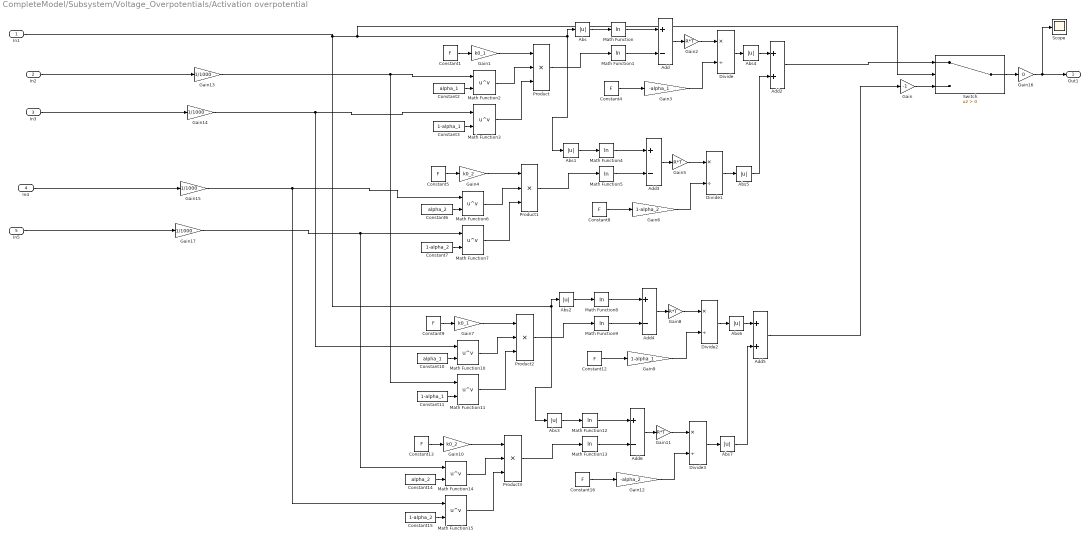
== system CompleteModel/Subsystem/Voltage_Overpotentials/Activation overpotential ==
  In1 : Inport
  In2 : Inport  Port=2
  In3 : Inport  Port=3
  In4 : Inport  Port=4
  In5 : Inport  Port=5
  Abs{,1..7} (8 alike) : Abs
  Add{,3..4,6} (4 alike) : Sum  Inputs=+-
  Add2 : Sum
  Add5 : Sum
  Constant{1,4..5,8..9,12..13,16} (8 alike) : Constant  Value=F
  Constant10 : Constant  Value=alpha_1
  Constant11 : Constant  Value=1-alpha_1
  Constant14 : Constant  Value=alpha_2
  Constant15 : Constant  Value=1-alpha_2
  Constant2 : Constant  Value=alpha_1
  Constant3 : Constant  Value=1-alpha_1
  Constant6 : Constant  Value=alpha_2
  Constant7 : Constant  Value=1-alpha_2
  Divide{,1..3} (4 alike) : Product  Inputs=*/
  Gain : Gain  Gain=-1
  Gain1 : Gain  Gain=k0_1
  Gain10 : Gain  Gain=k0_2
  Gain{2,5,8,11} (4 alike) : Gain  Gain=R*T
  Gain12 : Gain  Gain=-alpha_2
  Gain{13..15,17} (4 alike) : Gain  Gain=1/1000
  Gain16 : Gain  Gain=0
  Gain3 : Gain  Gain=-alpha_1
  Gain4 : Gain  Gain=k0_2
  Gain6 : Gain  Gain=1-alpha_2
  Gain7 : Gain  Gain=k0_1
  Gain9 : Gain  Gain=1-alpha_1
  Math Function{,1,4..5,8..9,12..13} (8 alike) : Math  Operator=log  SaturateOnIntegerOverflow=on
  Math Function{2..3,6..7,10..11,14..15} (8 alike) : Math  Operator=pow  SaturateOnIntegerOverflow=on
  Product{,1..3} (4 alike) : Product  Inputs=3
  Scope : Scope
  Switch : Switch  Criteria=u2 > Threshold
  Out1 : Outport
  wires:
  Divide/1 -> Abs4/1
  Constant1/1 -> Gain1/1
  Constant5/1 -> Gain4/1
  In5/1 -> Gain17/1
  Product1/1 -> Math Function5/1
  In1/1 -> Abs2/1, Abs3/1, Switch/2, Abs/1, Abs1/1
  Abs/1 -> Math Function/1
  Constant8/1 -> Gain6/1
  Constant2/1 -> Math Function2/2
  Math Function2/1 -> Product/2
  Gain5/1 -> Divide1/1
  Math Function5/1 -> Add3/2
  Add/1 -> Gain2/1
  Math Function4/1 -> Add3/1
  Gain12/1 -> Divide3/2
  Add6/1 -> Gain11/1
  Switch/1 -> Gain16/1
  Constant7/1 -> Math Function7/2
  Constant15/1 -> Math Function15/2
  Gain3/1 -> Divide/2
  Abs1/1 -> Math Function4/1
  Product3/1 -> Math Function13/1
  Add4/1 -> Gain8/1
  Math Function7/1 -> Product1/3
  In4/1 -> Gain15/1
  Constant3/1 -> Math Function3/2
  Product2/1 -> Math Function9/1
  Gain6/1 -> Divide1/2
  Gain8/1 -> Divide2/1
  Math Function6/1 -> Product1/2
  Constant14/1 -> Math Function14/2
  Gain4/1 -> Product1/1
  Constant6/1 -> Math Function6/2
  In3/1 -> Gain14/1
  Gain1/1 -> Product/1
  Math Function15/1 -> Product3/3
  Constant13/1 -> Gain10/1
  Gain11/1 -> Divide3/1
  Gain10/1 -> Product3/1
  Constant11/1 -> Math Function11/2
  Abs2/1 -> Math Function8/1
  Math Function8/1 -> Add4/1
  Product/1 -> Math Function1/1
  Constant12/1 -> Gain9/1
  Divide1/1 -> Abs5/1
  Math Function3/1 -> Product/3
  Gain9/1 -> Divide2/2
  Divide2/1 -> Abs6/1
  Gain7/1 -> Product2/1
  Gain2/1 -> Divide/1
  Constant4/1 -> Gain3/1
  Divide3/1 -> Abs7/1
  Math Function11/1 -> Product2/3
  Add3/1 -> Gain5/1
  Add5/1 -> Gain/1
  Abs3/1 -> Math Function12/1
  Constant10/1 -> Math Function10/2
  Math Function9/1 -> Add4/2
  Math Function14/1 -> Product3/2
  Math Function10/1 -> Product2/2
  Math Function13/1 -> Add6/2
  Math Function12/1 -> Add6/1
  Constant16/1 -> Gain12/1
  Constant9/1 -> Gain7/1
  In2/1 -> Gain13/1
  Math Function/1 -> Add/1
  Math Function1/1 -> Add/2
  Gain13/1 -> Math Function11/1, Math Function2/1
  Gain14/1 -> Math Function10/1, Math Function3/1
  Gain15/1 -> Math Function15/1, Math Function6/1
  Gain17/1 -> Math Function14/1, Math Function7/1
  Gain/1 -> Switch/3
  Add2/1 -> Switch/1
  Abs4/1 -> Add2/1
  Abs5/1 -> Add2/2
  Abs6/1 -> Add5/1
  Abs7/1 -> Add5/2
  Gain16/1 -> Scope/1, Out1/1

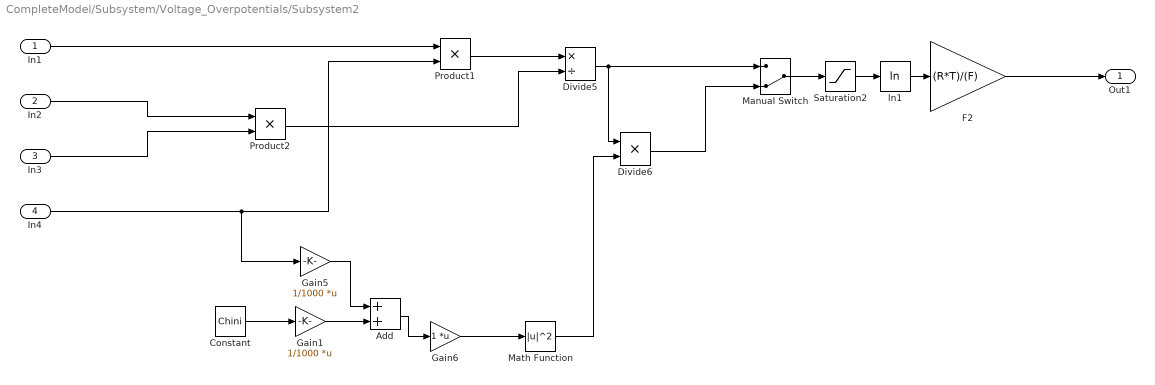
== system CompleteModel/Subsystem/Voltage_Overpotentials/Subsystem2 ==
  In1 : Inport
  In2 : Inport  Port=2
  In3 : Inport  Port=3
  In4 : Inport  Port=4
  Add : Sum
  Constant : Constant  Value=Chini
  Divide5 : Product  Inputs=*/
  Divide6 : Product  Inputs=**
  F2 : Gain  Gain=(R*T)/(F)
  Gain1 : Gain  Gain=1/1000  Multiplication=Matrix(K*u)
  Gain5 : Gain  Gain=1/1000  Multiplication=Matrix(K*u)
  Gain6 : Gain  Multiplication=Matrix(K*u)
  Manual Switch : ManualSwitch  CurrentSetting=0
  Math Function : Math  Operator=magnitude^2  SaturateOnIntegerOverflow=on
  Product1 : Product
  Product2 : Product
  Saturation2 : Saturate  UpperLimit=1e5  LowerLimit=1e-5
  ln1 : Math  Operator=log  SignedPower=on  SaturateOnIntegerOverflow=on
  Out1 : Outport
  wires:
  Gain5/1 -> Add/1
  Gain6/1 -> Math Function/1
  Manual Switch/1 -> Saturation2/1
  Product1/1 -> Divide5/1
  In3/1 -> Product2/2
  ln1/1 -> F2/1
  Divide6/1 -> Manual Switch/2
  Add/1 -> Gain6/1
  Divide5/1 -> Divide6/1, Manual Switch/1
  Constant/1 -> Gain1/1
  Saturation2/1 -> ln1/1
  In2/1 -> Product2/1
  In4/1 -> Gain5/1, Product1/2
  Math Function/1 -> Divide6/2
  Product2/1 -> Divide5/2
  F2/1 -> Out1/1
  In1/1 -> Product1/1
  Gain1/1 -> Add/2

== system CompleteModel/Subsystem/Hydraulic_pressure/Pressure_Losses_Line1/Elbows_Losses ==
  Q1 : Inport
  Gain1 : Gain  Gain=[1 1 1/3]
  Gain2 : Gain  Gain=4/pi
  Gain3 : Gain  Gain=1./(D_L1.^2)
  Gain4 : Gain  Gain=K_E1.*N_E1
  Gain5 : Gain  Gain=ro/2
  Product : Product
  Sum of Elements : Sum  Inputs=+
  Pelb : Outport  VectorParamsAs1DForOutWhenUnconnected=off
  Pelb_pipes : Outport  Port=2  VectorParamsAs1DForOutWhenUnconnected=off
  wires:
  Q1/1 -> Gain1/1
  Gain1/1 -> Gain2/1
  Gain2/1 -> Gain3/1
  Sum of Elements/1 -> Pelb/1
  Gain3/1 -> Product/2, Product/1
  Product/1 -> Gain4/1
  Gain4/1 -> Gain5/1
  Gain5/1 -> Sum of Elements/1, Pelb_pipes/1

== system CompleteModel/Subsystem/Hydraulic_pressure/Pressure_Losses_Line1/Flow_Division_Losses ==
  Q1 : Inport
  Demux : Demux  Outputs=3
  Gain1 : Gain  Gain=[1 1 1/3]
  Gain2 : Gain  Gain=4/pi
  Gain3 : Gain  Gain=1./(D_L1.^2)
  Gain4 : Gain  Gain=ro*(K_con1+K_exp1)/2
  Product2 : Product
  Pflow_div : Outport  VectorParamsAs1DForOutWhenUnconnected=off
  wires:
  Q1/1 -> Gain1/1
  Gain1/1 -> Gain2/1
  Gain2/1 -> Gain3/1
  Gain3/1 -> Demux/1
  Product2/1 -> Gain4/1
  Gain4/1 -> Pflow_div/1
  Demux/3 -> Product2/1, Product2/2

== system CompleteModel/Subsystem/Hydraulic_pressure/Pressure_Losses_Line1/Input_Output_Losses ==
  Q1 : Inport
  Add : Sum
  Demux : Demux  Outputs=3
  Gain1 : Gain  Gain=[1 1 1/3]
  Gain2 : Gain  Gain=4/pi
  Gain3 : Gain  Gain=1./(D_L1.^2)
  Gain4 : Gain  Gain=ro*K_out1*N_out1/2
  Gain5 : Gain  Gain=ro*K_in1*N_in1/2
  Product2 : Product
  Pin_out : Outport  VectorParamsAs1DForOutWhenUnconnected=off
  wires:
  Q1/1 -> Gain1/1
  Gain1/1 -> Gain2/1
  Gain2/1 -> Gain3/1
  Gain3/1 -> Demux/1
  Product2/1 -> Gain4/1, Gain5/1
  Add/1 -> Pin_out/1
  Demux/3 -> Product2/1, Product2/2
  Gain5/1 -> Add/1
  Gain4/1 -> Add/2

== system CompleteModel/Subsystem/Hydraulic_pressure/Pressure_Losses_Line1/Pipes_Distributed_Losses ==
  "Q1 " : Inport
  Gain1 : Gain  Gain=[1 1 1/3]
  Gain2 : Gain  Gain=4/pi
  Gain3 : Gain  Gain=1./(D_L1.^2)
  Gain4 : Gain  Gain=ro*f_L1.*L_L1./(2*D_L1)
  Product : Product
  Sum of Elements : Sum  Inputs=+
  Pdis_L1 : Outport  VectorParamsAs1DForOutWhenUnconnected=off
  Pdis_L1_pipes : Outport  Port=2  VectorParamsAs1DForOutWhenUnconnected=off
  wires:
  Gain2/1 -> Gain3/1
  "Q1 "/1 -> Gain1/1
  Sum of Elements/1 -> Pdis_L1/1
  Gain4/1 -> Pdis_L1_pipes/1, Sum of Elements/1
  Gain1/1 -> Gain2/1
  Gain3/1 -> Product/2, Product/1
  Product/1 -> Gain4/1

== system CompleteModel/Subsystem/Hydraulic_pressure/Pressure_Losses_Line1/Section_Change_Losses ==
  Q1 : Inport
  Add : Sum  Inputs=+-
  Add1 : Sum
  Demux : Demux  Outputs=3
  Gain1 : Gain  Gain=[1 1 1/3]
  Gain2 : Gain  Gain=4/pi
  Gain3 : Gain  Gain=1./(D_L1.^2)
  Gain4 : Gain  Gain=K_inc1*ro/2
  Gain5 : Gain  Gain=K_dec1*ro/2
  Product1 : Product
  Product2 : Product
  Psec_change : Outport  VectorParamsAs1DForOutWhenUnconnected=off
  wires:
  Q1/1 -> Gain1/1
  Gain1/1 -> Gain2/1
  Gain2/1 -> Gain3/1
  Gain3/1 -> Demux/1
  Demux/1 -> Add/1
  Demux/2 -> Product2/1, Product2/2, Add/2
  Add/1 -> Product1/1, Product1/2
  Product1/1 -> Gain4/1
  Product2/1 -> Gain5/1
  Gain5/1 -> Add1/2
  Gain4/1 -> Add1/1
  Add1/1 -> Psec_change/1

== system CompleteModel/Subsystem/Hydraulic_pressure/Pressure_Losses_Line1/Valves_Losses ==
  Q1 : Inport
  Demux : Demux  Outputs=3
  Gain1 : Gain  Gain=[1 1 1/3]
  Gain2 : Gain  Gain=4/pi
  Gain3 : Gain  Gain=1./(D_L1.^2)
  Gain4 : Gain  Gain=N_valves1*K_valve1*ro/2
  Product : Product
  Pval : Outport  VectorParamsAs1DForOutWhenUnconnected=off
  wires:
  Q1/1 -> Gain1/1
  Gain1/1 -> Gain2/1
  Gain2/1 -> Gain3/1
  Gain4/1 -> Pval/1
  Gain3/1 -> Demux/1
  Product/1 -> Gain4/1
  Demux/1 -> Product/2, Product/1

== system CompleteModel/Subsystem/Hydraulic_pressure/Pressure_Losses_Line2/Elbows_Losses ==
  Q2 : Inport
  Gain1 : Gain  Gain=[1 1 1/3]
  Gain2 : Gain  Gain=4/pi
  Gain3 : Gain  Gain=1./(D_L2.^2)
  Gain4 : Gain  Gain=K_E2.*N_E2
  Gain5 : Gain  Gain=ro/2
  Product : Product
  Sum of Elements : Sum  Inputs=+
  Pelb : Outport  VectorParamsAs1DForOutWhenUnconnected=off
  Pelb_pipes : Outport  Port=2  VectorParamsAs1DForOutWhenUnconnected=off
  wires:
  Q2/1 -> Gain1/1
  Gain1/1 -> Gain2/1
  Gain2/1 -> Gain3/1
  Sum of Elements/1 -> Pelb/1
  Gain3/1 -> Product/2, Product/1
  Product/1 -> Gain4/1
  Gain4/1 -> Gain5/1
  Gain5/1 -> Sum of Elements/1, Pelb_pipes/1

== system CompleteModel/Subsystem/Hydraulic_pressure/Pressure_Losses_Line2/Flow_Division_Losses ==
  Q2 : Inport
  Demux : Demux  Outputs=3
  Gain1 : Gain  Gain=[1 1 1/3]
  Gain2 : Gain  Gain=4/pi
  Gain3 : Gain  Gain=1./(D_L2.^2)
  Gain4 : Gain  Gain=ro*(K_con2+K_exp2)/2
  Product2 : Product
  Pflow_div : Outport  VectorParamsAs1DForOutWhenUnconnected=off
  wires:
  Q2/1 -> Gain1/1
  Gain1/1 -> Gain2/1
  Gain2/1 -> Gain3/1
  Gain3/1 -> Demux/1
  Product2/1 -> Gain4/1
  Gain4/1 -> Pflow_div/1
  Demux/3 -> Product2/1, Product2/2

== system CompleteModel/Subsystem/Hydraulic_pressure/Pressure_Losses_Line2/Input_Output_Losses ==
  Q2 : Inport
  Add : Sum
  Demux : Demux  Outputs=3
  Gain1 : Gain  Gain=[1 1 1/3]
  Gain2 : Gain  Gain=4/pi
  Gain3 : Gain  Gain=1./(D_L2.^2)
  Gain4 : Gain  Gain=ro*K_out2*N_out2/2
  Gain5 : Gain  Gain=ro*K_in2*N_in2/2
  Product2 : Product
  Pin_out : Outport  VectorParamsAs1DForOutWhenUnconnected=off
  wires:
  Q2/1 -> Gain1/1
  Gain1/1 -> Gain2/1
  Gain2/1 -> Gain3/1
  Gain3/1 -> Demux/1
  Product2/1 -> Gain4/1, Gain5/1
  Add/1 -> Pin_out/1
  Demux/3 -> Product2/1, Product2/2
  Gain5/1 -> Add/1
  Gain4/1 -> Add/2

== system CompleteModel/Subsystem/Hydraulic_pressure/Pressure_Losses_Line2/Pipes_Distributed_Losses ==
  Q2 : Inport
  Gain1 : Gain  Gain=[1 1 1/3]
  Gain2 : Gain  Gain=4/pi
  Gain3 : Gain  Gain=1./(D_L2.^2)
  Gain4 : Gain  Gain=ro*f_L2.*L_L2./(2*D_L2)
  Product : Product
  Sum of Elements : Sum  Inputs=+
  Pdis : Outport  VectorParamsAs1DForOutWhenUnconnected=off
  Pdis_pipes : Outport  Port=2  VectorParamsAs1DForOutWhenUnconnected=off
  wires:
  Gain2/1 -> Gain3/1
  Q2/1 -> Gain1/1
  Sum of Elements/1 -> Pdis/1
  Gain4/1 -> Pdis_pipes/1, Sum of Elements/1
  Gain1/1 -> Gain2/1
  Gain3/1 -> Product/2, Product/1
  Product/1 -> Gain4/1

== system CompleteModel/Subsystem/Hydraulic_pressure/Pressure_Losses_Line2/Section_Change_Losses ==
  Q2 : Inport
  Add : Sum  Inputs=+-
  Add1 : Sum
  Demux : Demux  Outputs=3
  Gain1 : Gain  Gain=[1 1 1/3]
  Gain2 : Gain  Gain=4/pi
  Gain3 : Gain  Gain=1./(D_L2.^2)
  Gain4 : Gain  Gain=K_inc2*ro/2
  Gain5 : Gain  Gain=K_dec2*ro/2
  Product1 : Product
  Product2 : Product
  Psec_change : Outport  VectorParamsAs1DForOutWhenUnconnected=off
  wires:
  Q2/1 -> Gain1/1
  Gain1/1 -> Gain2/1
  Gain2/1 -> Gain3/1
  Gain3/1 -> Demux/1
  Demux/1 -> Add/1
  Demux/2 -> Product2/1, Product2/2, Add/2
  Add/1 -> Product1/1, Product1/2
  Product1/1 -> Gain4/1
  Product2/1 -> Gain5/1
  Gain5/1 -> Add1/2
  Gain4/1 -> Add1/1
  Add1/1 -> Psec_change/1

== system CompleteModel/Subsystem/Hydraulic_pressure/Pressure_Losses_Line2/Valves_Losses ==
  Q2 : Inport
  Demux : Demux  Outputs=3
  Gain1 : Gain  Gain=[1 1 1/3]
  Gain2 : Gain  Gain=4/pi
  Gain3 : Gain  Gain=1./(D_L2.^2)
  Gain4 : Gain  Gain=N_valves2*K_valve2*ro/2
  Product : Product
  Pval : Outport  VectorParamsAs1DForOutWhenUnconnected=off
  wires:
  Q2/1 -> Gain1/1
  Gain1/1 -> Gain2/1
  Gain2/1 -> Gain3/1
  Gain4/1 -> Pval/1
  Gain3/1 -> Demux/1
  Product/1 -> Gain4/1
  Demux/1 -> Product/2, Product/1

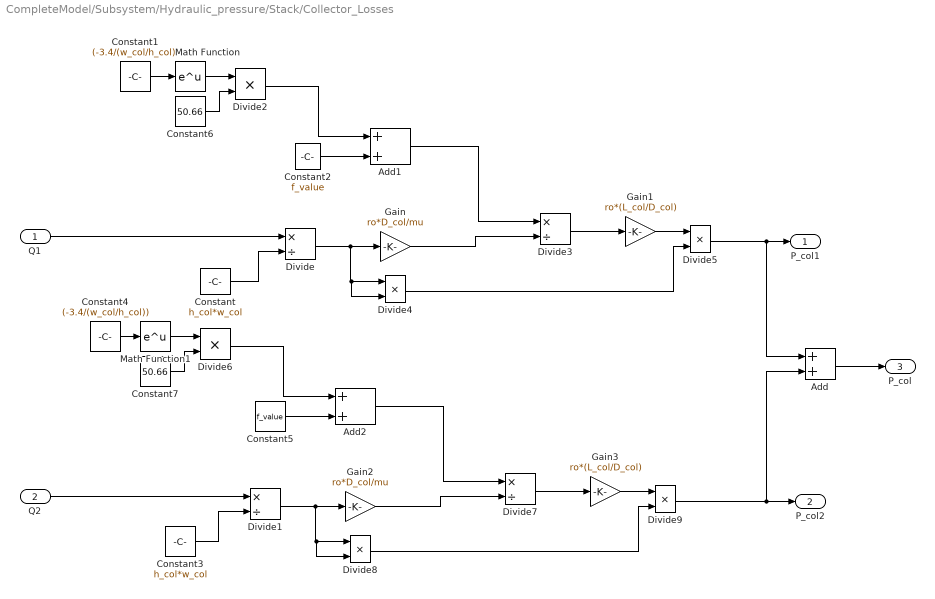
== system CompleteModel/Subsystem/Hydraulic_pressure/Stack/Collector_Losses ==
  Q1 : Inport
  Q2 : Inport  Port=2
  Add : Sum
  Add1 : Sum
  Add2 : Sum
  Constant : Constant  Value=h_col*w_col
  Constant1 : Constant  Value=(-3.4/(w_col/h_col))
  Constant2 : Constant  Value=f_value
  Constant3 : Constant  Value=h_col*w_col
  Constant4 : Constant  Value=(-3.4/(w_col/h_col))
  Constant5 : Constant  Value=f_value
  Constant6 : Constant  Value=50.66
  Constant7 : Constant  Value=50.66
  Divide{,1,3,7} (4 alike) : Product  Inputs=*/
  Divide{2,4..6,8..9} (6 alike) : Product  Inputs=**
  Gain : Gain  Gain=ro*D_col/mu
  Gain1 : Gain  Gain=ro*(L_col/D_col)
  Gain2 : Gain  Gain=ro*D_col/mu
  Gain3 : Gain  Gain=ro*(L_col/D_col)
  Math Function : Math  SignedPower=on  SaturateOnIntegerOverflow=on
  Math Function1 : Math  SignedPower=on  SaturateOnIntegerOverflow=on
  P_col1 : Outport  VectorParamsAs1DForOutWhenUnconnected=off
  P_col2 : Outport  Port=2  VectorParamsAs1DForOutWhenUnconnected=off
  P_col : Outport  Port=3  VectorParamsAs1DForOutWhenUnconnected=off
  wires:
  Q1/1 -> Divide/1
  Constant/1 -> Divide/2
  Divide/1 -> Divide4/2, Divide4/1, Gain/1
  Constant1/1 -> Math Function/1
  Math Function/1 -> Divide2/1
  Gain/1 -> Divide3/2
  Add1/1 -> Divide3/1
  Divide3/1 -> Gain1/1
  Divide4/1 -> Divide5/2
  Gain1/1 -> Divide5/1
  Divide5/1 -> Add/1, P_col1/1
  Add/1 -> P_col/1
  Constant2/1 -> Add1/2
  Divide2/1 -> Add1/1
  Constant6/1 -> Divide2/2
  Constant3/1 -> Divide1/2
  Divide6/1 -> Add2/1
  Divide8/1 -> Divide9/2
  Constant7/1 -> Divide6/2
  Gain2/1 -> Divide7/2
  Constant5/1 -> Add2/2
  Gain3/1 -> Divide9/1
  Q2/1 -> Divide1/1
  Constant4/1 -> Math Function1/1
  Divide9/1 -> P_col2/1, Add/2
  Math Function1/1 -> Divide6/1
  Add2/1 -> Divide7/1
  Divide7/1 -> Gain3/1
  Divide1/1 -> Divide8/2, Divide8/1, Gain2/1

== system CompleteModel/Subsystem/Hydraulic_pressure/Stack/Electrode_Losses ==
  Q1 : Inport
  Q2 : Inport  Port=2
  Add : Sum
  Constant1 : Constant  Value=K_el
  Constant2 : Constant  Value=K_el
  Divide1 : Product  Inputs=*/
  Divide2 : Product  Inputs=*/
  Gain1 : Gain  Gain=1/2
  Gain2 : Gain  Gain=1/2
  Gain3 : Gain  Gain=mu*L_el
  Gain4 : Gain  Gain=mu*L_el
  Gain5 : Gain  Gain=1/N
  Gain6 : Gain  Gain=1/N
  P_el1 : Outport  VectorParamsAs1DForOutWhenUnconnected=off
  P_el2 : Outport  Port=2  VectorParamsAs1DForOutWhenUnconnected=off
  P_el : Outport  Port=3  VectorParamsAs1DForOutWhenUnconnected=off
  wires:
  Q1/1 -> Gain5/1
  Add/1 -> P_el/1
  Gain1/1 -> P_el1/1, Add/1
  Gain2/1 -> Add/2, P_el2/1
  Gain4/1 -> Divide2/1
  Divide2/1 -> Gain1/1
  Q2/1 -> Gain6/1
  Divide1/1 -> Gain2/1
  Constant2/1 -> Divide1/2
  Gain3/1 -> Divide1/1
  Constant1/1 -> Divide2/2
  Gain5/1 -> Gain4/1
  Gain6/1 -> Gain3/1
